simulink model "BMS"  (R2024b)
settings: Solver=ode23tb  StartTime=0.0  StopTime=1  RelTol=1e-3  EnableMultiTasking=on
PreLoadFcn:
  | % Data of Solar Panel
  | %5000[W]/130[W]
  | % Total power generated by solar panel reaches 5[KW].
  | % each solar panel generates power 130[kW].
  | V = [0    40 80 120 160 180 200 217 240 260 280];
  | I = 5000/130*[0.68 0.675 0.67 0.665 0.660 0.655 0.640 0.6 0.48 0.28 0];
  | 
  | %subplot(211);plot(V,I);xlabel('Voltage[V]');ylabel('Current[a]')
  | %subplot(212);plot(V.*I);title('Power[W]')
  | 
  | % Sample Time[s]
  | Ts =5e-6;
  | 
  | 
  | %MPPT + PV Control
  | % PI control pamameter of Voltage control(Outer loop)
  | Kp_V = 50e-3;
  | Ki_V = 10;
  | 
  | % PI Control pamameter of Current control(Inner loop)
  | Kp_I = 25e-3;
  | Ki_I = 10;
  | 
  | % Utility Interconnection Control
  | % PI Control pamameter of Voltage control(Outer loop)
  | Kp_V2 = 0.01;
  | Ki_V2 = 25;
  | 
  | % PI control pamameter of Current control(Inner loop)
  | Kp_I2 = 0.01;
  | Ki_I2 = 25;
  | 
  | 
  | % Difference of voltege using in MPPT
  | dV = 0.5;
  | 
  | % Battery Control
  | % PI Control pamameter of Voltage control(Outer loop)
  | Kp_VB = 0.4;
  | Ki_VB = 2;
  | 
  | % PI control pamameter of Current control(Inner loop)
  | Kp_IB = 0.1;
  | Ki_IB = 0.5;
undefined symbols (not defined in the file): Acid, Ion, Lead, Lithium, sigbuilder_block
libraries: spsBreakerLib x120, spsBatteryLib x111, spsSeriesRLCBranchLib x59, spsVoltageMeasurementLib x17, spsIdealSwitchLib x15, spsMosfetLib x11, slpidlib x9, spsCurrentMeasurementLib x7, spsPWMGeneratorDCDCLib x7, spsDiodeLib x6, spsPWMGenerator2LevelLib x5, spspowerguiLib x3
(part 5 of 6)

== matlab function BMS/Subsystem18/Swapping battery controller/MATLAB Function7 ==
  settings: updateMethod=DISCRETE
  data: SOC input; LoadOn output; ChargingOn output
function [LoadOn, ChargingOn] = chargeDischargeNode(SOC)
    % This function determines the charging and discharging states
    % based on the state of charge (SOC) of the battery.
    % Inputs:
    %   SOC - Current state of charge (0 to 100)
    % Outputs:
    %   LoadOn - Indicator if the load is on (1) or off (0)
    %   ChargingOn - Indicator if charging is active (1) or not (0)

    % Initialize persistent variables to retain state across function calls
    persistent LoadOnPersistent;
    persistent ChargingOnPersistent;

    if isempty(LoadOnPersistent)  % Initialize on first call
        LoadOnPersistent = 1;     % Load is initially on
        ChargingOnPersistent = 0;  % Charging is initially off
    end

    % Logic for charging and discharging based on SOC levels
    if SOC > 80
        LoadOnPersistent = 1;      % Turn load on if SOC is above 80%
        ChargingOnPersistent = 0;   % Turn charging off
    elseif SOC < 40
        LoadOnPersistent = 0;      % Turn load off if SOC is below 40%
        ChargingOnPersistent = 1;   % Start charging
    end

    % Assign output values from persistent variables
    LoadOn = LoadOnPersistent;
    ChargingOn = ChargingOnPersistent;
end

== matlab function BMS/Subsystem18/Swapping battery controller/MATLAB Function8 ==
  settings: updateMethod=DISCRETE
  data: SOC input; LoadOn output; ChargingOn output
function [LoadOn, ChargingOn] = chargeDischargeNode(SOC)
    % This function determines the charging and discharging states
    % based on the state of charge (SOC) of the battery.
    % Inputs:
    %   SOC - Current state of charge (0 to 100)
    % Outputs:
    %   LoadOn - Indicator if the load is on (1) or off (0)
    %   ChargingOn - Indicator if charging is active (1) or not (0)

    % Initialize persistent variables to retain state across function calls
    persistent LoadOnPersistent;
    persistent ChargingOnPersistent;

    if isempty(LoadOnPersistent)  % Initialize on first call
        LoadOnPersistent = 1;     % Load is initially on
        ChargingOnPersistent = 0;  % Charging is initially off
    end

    % Logic for charging and discharging based on SOC levels
    if SOC > 80
        LoadOnPersistent = 1;      % Turn load on if SOC is above 80%
        ChargingOnPersistent = 0;   % Turn charging off
    elseif SOC < 40
        LoadOnPersistent = 0;      % Turn load off if SOC is below 40%
        ChargingOnPersistent = 1;   % Start charging
    end

    % Assign output values from persistent variables
    LoadOn = LoadOnPersistent;
    ChargingOn = ChargingOnPersistent;
end

== matlab function BMS/Subsystem18/Swapping battery controller/MATLAB Function9 ==
  settings: updateMethod=DISCRETE
  data: SOC input; LoadOn output; ChargingOn output
function [LoadOn, ChargingOn] = chargeDischargeNode(SOC)
    % This function determines the charging and discharging states
    % based on the state of charge (SOC) of the battery.
    % Inputs:
    %   SOC - Current state of charge (0 to 100)
    % Outputs:
    %   LoadOn - Indicator if the load is on (1) or off (0)
    %   ChargingOn - Indicator if charging is active (1) or not (0)

    % Initialize persistent variables to retain state across function calls
    persistent LoadOnPersistent;
    persistent ChargingOnPersistent;

    if isempty(LoadOnPersistent)  % Initialize on first call
        LoadOnPersistent = 1;     % Load is initially on
        ChargingOnPersistent = 0;  % Charging is initially off
    end

    % Logic for charging and discharging based on SOC levels
    if SOC > 80
        LoadOnPersistent = 1;      % Turn load on if SOC is above 80%
        ChargingOnPersistent = 0;   % Turn charging off
    elseif SOC < 40
        LoadOnPersistent = 0;      % Turn load off if SOC is below 40%
        ChargingOnPersistent = 1;   % Start charging
    end

    % Assign output values from persistent variables
    LoadOn = LoadOnPersistent;
    ChargingOn = ChargingOnPersistent;
end

== matlab function BMS/Subsystem18/Swapping battery controller/MATLAB Function10 ==
  settings: updateMethod=DISCRETE
  data: SOC input; LoadOn output; ChargingOn output
function [LoadOn, ChargingOn] = chargeDischargeNode(SOC)
    % This function determines the charging and discharging states
    % based on the state of charge (SOC) of the battery.
    % Inputs:
    %   SOC - Current state of charge (0 to 100)
    % Outputs:
    %   LoadOn - Indicator if the load is on (1) or off (0)
    %   ChargingOn - Indicator if charging is active (1) or not (0)

    % Initialize persistent variables to retain state across function calls
    persistent LoadOnPersistent;
    persistent ChargingOnPersistent;

    if isempty(LoadOnPersistent)  % Initialize on first call
        LoadOnPersistent = 1;     % Load is initially on
        ChargingOnPersistent = 0;  % Charging is initially off
    end

    % Logic for charging and discharging based on SOC levels
    if SOC > 80
        LoadOnPersistent = 1;      % Turn load on if SOC is above 80%
        ChargingOnPersistent = 0;   % Turn charging off
    elseif SOC < 40
        LoadOnPersistent = 0;      % Turn load off if SOC is below 40%
        ChargingOnPersistent = 1;   % Start charging
    end

    % Assign output values from persistent variables
    LoadOn = LoadOnPersistent;
    ChargingOn = ChargingOnPersistent;
end

== matlab function BMS/Subsystem18/Swapping battery controller/MATLAB Function11 ==
  settings: updateMethod=DISCRETE
  data: SOC input; LoadOn output; ChargingOn output
function [LoadOn, ChargingOn] = chargeDischargeNode(SOC)
    % This function determines the charging and discharging states
    % based on the state of charge (SOC) of the battery.
    % Inputs:
    %   SOC - Current state of charge (0 to 100)
    % Outputs:
    %   LoadOn - Indicator if the load is on (1) or off (0)
    %   ChargingOn - Indicator if charging is active (1) or not (0)

    % Initialize persistent variables to retain state across function calls
    persistent LoadOnPersistent;
    persistent ChargingOnPersistent;

    if isempty(LoadOnPersistent)  % Initialize on first call
        LoadOnPersistent = 1;     % Load is initially on
        ChargingOnPersistent = 0;  % Charging is initially off
    end

    % Logic for charging and discharging based on SOC levels
    if SOC > 80
        LoadOnPersistent = 1;      % Turn load on if SOC is above 80%
        ChargingOnPersistent = 0;   % Turn charging off
    elseif SOC < 40
        LoadOnPersistent = 0;      % Turn load off if SOC is below 40%
        ChargingOnPersistent = 1;   % Start charging
    end

    % Assign output values from persistent variables
    LoadOn = LoadOnPersistent;
    ChargingOn = ChargingOnPersistent;
end

== matlab function BMS/Subsystem18/Swapping battery controller/MATLAB Function12 ==
  settings: updateMethod=DISCRETE
  data: SOC input; LoadOn output; ChargingOn output
function [LoadOn, ChargingOn] = chargeDischargeNode(SOC)
    % This function determines the charging and discharging states
    % based on the state of charge (SOC) of the battery.
    % Inputs:
    %   SOC - Current state of charge (0 to 100)
    % Outputs:
    %   LoadOn - Indicator if the load is on (1) or off (0)
    %   ChargingOn - Indicator if charging is active (1) or not (0)

    % Initialize persistent variables to retain state across function calls
    persistent LoadOnPersistent;
    persistent ChargingOnPersistent;

    if isempty(LoadOnPersistent)  % Initialize on first call
        LoadOnPersistent = 1;     % Load is initially on
        ChargingOnPersistent = 0;  % Charging is initially off
    end

    % Logic for charging and discharging based on SOC levels
    if SOC > 80
        LoadOnPersistent = 1;      % Turn load on if SOC is above 80%
        ChargingOnPersistent = 0;   % Turn charging off
    elseif SOC < 40
        LoadOnPersistent = 0;      % Turn load off if SOC is below 40%
        ChargingOnPersistent = 1;   % Start charging
    end

    % Assign output values from persistent variables
    LoadOn = LoadOnPersistent;
    ChargingOn = ChargingOnPersistent;
end

== matlab function BMS/Subsystem18/Swapping battery controller/MATLAB Function13 ==
  settings: updateMethod=DISCRETE
  data: SOC input; LoadOn output; ChargingOn output
function [LoadOn, ChargingOn] = chargeDischargeNode(SOC)
    % This function determines the charging and discharging states
    % based on the state of charge (SOC) of the battery.
    % Inputs:
    %   SOC - Current state of charge (0 to 100)
    % Outputs:
    %   LoadOn - Indicator if the load is on (1) or off (0)
    %   ChargingOn - Indicator if charging is active (1) or not (0)

    % Initialize persistent variables to retain state across function calls
    persistent LoadOnPersistent;
    persistent ChargingOnPersistent;

    if isempty(LoadOnPersistent)  % Initialize on first call
        LoadOnPersistent = 1;     % Load is initially on
        ChargingOnPersistent = 0;  % Charging is initially off
    end

    % Logic for charging and discharging based on SOC levels
    if SOC > 80
        LoadOnPersistent = 1;      % Turn load on if SOC is above 80%
        ChargingOnPersistent = 0;   % Turn charging off
    elseif SOC < 40
        LoadOnPersistent = 0;      % Turn load off if SOC is below 40%
        ChargingOnPersistent = 1;   % Start charging
    end

    % Assign output values from persistent variables
    LoadOn = LoadOnPersistent;
    ChargingOn = ChargingOnPersistent;
end

== matlab function BMS/Subsystem18/Swapping battery controller/MATLAB Function14 ==
  settings: updateMethod=DISCRETE
  data: SOC input; LoadOn output; ChargingOn output
function [LoadOn, ChargingOn] = chargeDischargeNode(SOC)
    % This function determines the charging and discharging states
    % based on the state of charge (SOC) of the battery.
    % Inputs:
    %   SOC - Current state of charge (0 to 100)
    % Outputs:
    %   LoadOn - Indicator if the load is on (1) or off (0)
    %   ChargingOn - Indicator if charging is active (1) or not (0)

    % Initialize persistent variables to retain state across function calls
    persistent LoadOnPersistent;
    persistent ChargingOnPersistent;

    if isempty(LoadOnPersistent)  % Initialize on first call
        LoadOnPersistent = 1;     % Load is initially on
        ChargingOnPersistent = 0;  % Charging is initially off
    end

    % Logic for charging and discharging based on SOC levels
    if SOC > 80
        LoadOnPersistent = 1;      % Turn load on if SOC is above 80%
        ChargingOnPersistent = 0;   % Turn charging off
    elseif SOC < 40
        LoadOnPersistent = 0;      % Turn load off if SOC is below 40%
        ChargingOnPersistent = 1;   % Start charging
    end

    % Assign output values from persistent variables
    LoadOn = LoadOnPersistent;
    ChargingOn = ChargingOnPersistent;
end

== matlab function BMS/Subsystem18/Swapping battery controller/MATLAB Function15 ==
  settings: updateMethod=DISCRETE
  data: SOC input; LoadOn output; ChargingOn output
function [LoadOn, ChargingOn] = chargeDischargeNode(SOC)
    % This function determines the charging and discharging states
    % based on the state of charge (SOC) of the battery.
    % Inputs:
    %   SOC - Current state of charge (0 to 100)
    % Outputs:
    %   LoadOn - Indicator if the load is on (1) or off (0)
    %   ChargingOn - Indicator if charging is active (1) or not (0)

    % Initialize persistent variables to retain state across function calls
    persistent LoadOnPersistent;
    persistent ChargingOnPersistent;

    if isempty(LoadOnPersistent)  % Initialize on first call
        LoadOnPersistent = 1;     % Load is initially on
        ChargingOnPersistent = 0;  % Charging is initially off
    end

    % Logic for charging and discharging based on SOC levels
    if SOC > 80
        LoadOnPersistent = 1;      % Turn load on if SOC is above 80%
        ChargingOnPersistent = 0;   % Turn charging off
    elseif SOC < 40
        LoadOnPersistent = 0;      % Turn load off if SOC is below 40%
        ChargingOnPersistent = 1;   % Start charging
    end

    % Assign output values from persistent variables
    LoadOn = LoadOnPersistent;
    ChargingOn = ChargingOnPersistent;
end

== matlab function BMS/Subsystem18/Swapping battery controller/MATLAB Function16 ==
  settings: updateMethod=DISCRETE
  data: SOC input; LoadOn output; ChargingOn output
function [LoadOn, ChargingOn] = chargeDischargeNode(SOC)
    % This function determines the charging and discharging states
    % based on the state of charge (SOC) of the battery.
    % Inputs:
    %   SOC - Current state of charge (0 to 100)
    % Outputs:
    %   LoadOn - Indicator if the load is on (1) or off (0)
    %   ChargingOn - Indicator if charging is active (1) or not (0)

    % Initialize persistent variables to retain state across function calls
    persistent LoadOnPersistent;
    persistent ChargingOnPersistent;

    if isempty(LoadOnPersistent)  % Initialize on first call
        LoadOnPersistent = 1;     % Load is initially on
        ChargingOnPersistent = 0;  % Charging is initially off
    end

    % Logic for charging and discharging based on SOC levels
    if SOC > 80
        LoadOnPersistent = 1;      % Turn load on if SOC is above 80%
        ChargingOnPersistent = 0;   % Turn charging off
    elseif SOC < 40
        LoadOnPersistent = 0;      % Turn load off if SOC is below 40%
        ChargingOnPersistent = 1;   % Start charging
    end

    % Assign output values from persistent variables
    LoadOn = LoadOnPersistent;
    ChargingOn = ChargingOnPersistent;
end

== matlab function BMS/Subsystem18/Swapping battery controller/MATLAB Function17 ==
  settings: updateMethod=DISCRETE
  data: SOC input; LoadOn output; ChargingOn output
function [LoadOn, ChargingOn] = chargeDischargeNode(SOC)
    % This function determines the charging and discharging states
    % based on the state of charge (SOC) of the battery.
    % Inputs:
    %   SOC - Current state of charge (0 to 100)
    % Outputs:
    %   LoadOn - Indicator if the load is on (1) or off (0)
    %   ChargingOn - Indicator if charging is active (1) or not (0)

    % Initialize persistent variables to retain state across function calls
    persistent LoadOnPersistent;
    persistent ChargingOnPersistent;

    if isempty(LoadOnPersistent)  % Initialize on first call
        LoadOnPersistent = 1;     % Load is initially on
        ChargingOnPersistent = 0;  % Charging is initially off
    end

    % Logic for charging and discharging based on SOC levels
    if SOC > 80
        LoadOnPersistent = 1;      % Turn load on if SOC is above 80%
        ChargingOnPersistent = 0;   % Turn charging off
    elseif SOC < 40
        LoadOnPersistent = 0;      % Turn load off if SOC is below 40%
        ChargingOnPersistent = 1;   % Start charging
    end

    % Assign output values from persistent variables
    LoadOn = LoadOnPersistent;
    ChargingOn = ChargingOnPersistent;
end

== matlab function BMS/Subsystem18/Swapping battery controller/MATLAB Function18 ==
  settings: updateMethod=DISCRETE
  data: SOC input; LoadOn output; ChargingOn output
function [LoadOn, ChargingOn] = chargeDischargeNode(SOC)
    % This function determines the charging and discharging states
    % based on the state of charge (SOC) of the battery.
    % Inputs:
    %   SOC - Current state of charge (0 to 100)
    % Outputs:
    %   LoadOn - Indicator if the load is on (1) or off (0)
    %   ChargingOn - Indicator if charging is active (1) or not (0)

    % Initialize persistent variables to retain state across function calls
    persistent LoadOnPersistent;
    persistent ChargingOnPersistent;

    if isempty(LoadOnPersistent)  % Initialize on first call
        LoadOnPersistent = 1;     % Load is initially on
        ChargingOnPersistent = 0;  % Charging is initially off
    end

    % Logic for charging and discharging based on SOC levels
    if SOC > 80
        LoadOnPersistent = 1;      % Turn load on if SOC is above 80%
        ChargingOnPersistent = 0;   % Turn charging off
    elseif SOC < 40
        LoadOnPersistent = 0;      % Turn load off if SOC is below 40%
        ChargingOnPersistent = 1;   % Start charging
    end

    % Assign output values from persistent variables
    LoadOn = LoadOnPersistent;
    ChargingOn = ChargingOnPersistent;
end

== matlab function BMS/Subsystem18/Swapping battery controller/MATLAB Function19 ==
  settings: updateMethod=DISCRETE
  data: SOC input; LoadOn output; ChargingOn output
function [LoadOn, ChargingOn] = chargeDischargeNode(SOC)
    % This function determines the charging and discharging states
    % based on the state of charge (SOC) of the battery.
    % Inputs:
    %   SOC - Current state of charge (0 to 100)
    % Outputs:
    %   LoadOn - Indicator if the load is on (1) or off (0)
    %   ChargingOn - Indicator if charging is active (1) or not (0)

    % Initialize persistent variables to retain state across function calls
    persistent LoadOnPersistent;
    persistent ChargingOnPersistent;

    if isempty(LoadOnPersistent)  % Initialize on first call
        LoadOnPersistent = 1;     % Load is initially on
        ChargingOnPersistent = 0;  % Charging is initially off
    end

    % Logic for charging and discharging based on SOC levels
    if SOC > 80
        LoadOnPersistent = 1;      % Turn load on if SOC is above 80%
        ChargingOnPersistent = 0;   % Turn charging off
    elseif SOC < 40
        LoadOnPersistent = 0;      % Turn load off if SOC is below 40%
        ChargingOnPersistent = 1;   % Start charging
    end

    % Assign output values from persistent variables
    LoadOn = LoadOnPersistent;
    ChargingOn = ChargingOnPersistent;
end

== matlab function BMS/Subsystem18/Swapping battery controller/MATLAB Function20 ==
  settings: updateMethod=DISCRETE
  data: SOC input; LoadOn output; ChargingOn output
function [LoadOn, ChargingOn] = chargeDischargeNode(SOC)
    % This function determines the charging and discharging states
    % based on the state of charge (SOC) of the battery.
    % Inputs:
    %   SOC - Current state of charge (0 to 100)
    % Outputs:
    %   LoadOn - Indicator if the load is on (1) or off (0)
    %   ChargingOn - Indicator if charging is active (1) or not (0)

    % Initialize persistent variables to retain state across function calls
    persistent LoadOnPersistent;
    persistent ChargingOnPersistent;

    if isempty(LoadOnPersistent)  % Initialize on first call
        LoadOnPersistent = 1;     % Load is initially on
        ChargingOnPersistent = 0;  % Charging is initially off
    end

    % Logic for charging and discharging based on SOC levels
    if SOC > 80
        LoadOnPersistent = 1;      % Turn load on if SOC is above 80%
        ChargingOnPersistent = 0;   % Turn charging off
    elseif SOC < 40
        LoadOnPersistent = 0;      % Turn load off if SOC is below 40%
        ChargingOnPersistent = 1;   % Start charging
    end

    % Assign output values from persistent variables
    LoadOn = LoadOnPersistent;
    ChargingOn = ChargingOnPersistent;
end

== matlab function BMS/Subsystem18/Swapping battery controller/MATLAB Function21 ==
  settings: updateMethod=DISCRETE
  data: SOC input; LoadOn output; ChargingOn output
function [LoadOn, ChargingOn] = chargeDischargeNode(SOC)
    % This function determines the charging and discharging states
    % based on the state of charge (SOC) of the battery.
    % Inputs:
    %   SOC - Current state of charge (0 to 100)
    % Outputs:
    %   LoadOn - Indicator if the load is on (1) or off (0)
    %   ChargingOn - Indicator if charging is active (1) or not (0)

    % Initialize persistent variables to retain state across function calls
    persistent LoadOnPersistent;
    persistent ChargingOnPersistent;

    if isempty(LoadOnPersistent)  % Initialize on first call
        LoadOnPersistent = 1;     % Load is initially on
        ChargingOnPersistent = 0;  % Charging is initially off
    end

    % Logic for charging and discharging based on SOC levels
    if SOC > 80
        LoadOnPersistent = 1;      % Turn load on if SOC is above 80%
        ChargingOnPersistent = 0;   % Turn charging off
    elseif SOC < 40
        LoadOnPersistent = 0;      % Turn load off if SOC is below 40%
        ChargingOnPersistent = 1;   % Start charging
    end

    % Assign output values from persistent variables
    LoadOn = LoadOnPersistent;
    ChargingOn = ChargingOnPersistent;
end

== matlab function BMS/Subsystem18/Swapping battery controller/MATLAB Function22 ==
  settings: updateMethod=DISCRETE
  data: SOC input; LoadOn output; ChargingOn output
function [LoadOn, ChargingOn] = chargeDischargeNode(SOC)
    % This function determines the charging and discharging states
    % based on the state of charge (SOC) of the battery.
    % Inputs:
    %   SOC - Current state of charge (0 to 100)
    % Outputs:
    %   LoadOn - Indicator if the load is on (1) or off (0)
    %   ChargingOn - Indicator if charging is active (1) or not (0)

    % Initialize persistent variables to retain state across function calls
    persistent LoadOnPersistent;
    persistent ChargingOnPersistent;

    if isempty(LoadOnPersistent)  % Initialize on first call
        LoadOnPersistent = 1;     % Load is initially on
        ChargingOnPersistent = 0;  % Charging is initially off
    end

    % Logic for charging and discharging based on SOC levels
    if SOC > 80
        LoadOnPersistent = 1;      % Turn load on if SOC is above 80%
        ChargingOnPersistent = 0;   % Turn charging off
    elseif SOC < 40
        LoadOnPersistent = 0;      % Turn load off if SOC is below 40%
        ChargingOnPersistent = 1;   % Start charging
    end

    % Assign output values from persistent variables
    LoadOn = LoadOnPersistent;
    ChargingOn = ChargingOnPersistent;
end

== matlab function BMS/Subsystem18/Swapping battery controller/MATLAB Function23 ==
  settings: updateMethod=DISCRETE
  data: SOC input; LoadOn output; ChargingOn output
function [LoadOn, ChargingOn] = chargeDischargeNode(SOC)
    % This function determines the charging and discharging states
    % based on the state of charge (SOC) of the battery.
    % Inputs:
    %   SOC - Current state of charge (0 to 100)
    % Outputs:
    %   LoadOn - Indicator if the load is on (1) or off (0)
    %   ChargingOn - Indicator if charging is active (1) or not (0)

    % Initialize persistent variables to retain state across function calls
    persistent LoadOnPersistent;
    persistent ChargingOnPersistent;

    if isempty(LoadOnPersistent)  % Initialize on first call
        LoadOnPersistent = 1;     % Load is initially on
        ChargingOnPersistent = 0;  % Charging is initially off
    end

    % Logic for charging and discharging based on SOC levels
    if SOC > 80
        LoadOnPersistent = 1;      % Turn load on if SOC is above 80%
        ChargingOnPersistent = 0;   % Turn charging off
    elseif SOC < 40
        LoadOnPersistent = 0;      % Turn load off if SOC is below 40%
        ChargingOnPersistent = 1;   % Start charging
    end

    % Assign output values from persistent variables
    LoadOn = LoadOnPersistent;
    ChargingOn = ChargingOnPersistent;
end

== matlab function BMS/Subsystem18/Swapping battery controller/MATLAB Function24 ==
  settings: updateMethod=DISCRETE
  data: SOC input; LoadOn output; ChargingOn output
function [LoadOn, ChargingOn] = chargeDischargeNode(SOC)
    % This function determines the charging and discharging states
    % based on the state of charge (SOC) of the battery.
    % Inputs:
    %   SOC - Current state of charge (0 to 100)
    % Outputs:
    %   LoadOn - Indicator if the load is on (1) or off (0)
    %   ChargingOn - Indicator if charging is active (1) or not (0)

    % Initialize persistent variables to retain state across function calls
    persistent LoadOnPersistent;
    persistent ChargingOnPersistent;

    if isempty(LoadOnPersistent)  % Initialize on first call
        LoadOnPersistent = 1;     % Load is initially on
        ChargingOnPersistent = 0;  % Charging is initially off
    end

    % Logic for charging and discharging based on SOC levels
    if SOC > 80
        LoadOnPersistent = 1;      % Turn load on if SOC is above 80%
        ChargingOnPersistent = 0;   % Turn charging off
    elseif SOC < 40
        LoadOnPersistent = 0;      % Turn load off if SOC is below 40%
        ChargingOnPersistent = 1;   % Start charging
    end

    % Assign output values from persistent variables
    LoadOn = LoadOnPersistent;
    ChargingOn = ChargingOnPersistent;
end

== matlab function BMS/Subsystem18/Swapping battery controller/MATLAB Function25 ==
  settings: updateMethod=DISCRETE
  data: SOC input; LoadOn output; ChargingOn output
function [LoadOn, ChargingOn] = chargeDischargeNode(SOC)
    % This function determines the charging and discharging states
    % based on the state of charge (SOC) of the battery.
    % Inputs:
    %   SOC - Current state of charge (0 to 100)
    % Outputs:
    %   LoadOn - Indicator if the load is on (1) or off (0)
    %   ChargingOn - Indicator if charging is active (1) or not (0)

    % Initialize persistent variables to retain state across function calls
    persistent LoadOnPersistent;
    persistent ChargingOnPersistent;

    if isempty(LoadOnPersistent)  % Initialize on first call
        LoadOnPersistent = 1;     % Load is initially on
        ChargingOnPersistent = 0;  % Charging is initially off
    end

    % Logic for charging and discharging based on SOC levels
    if SOC > 80
        LoadOnPersistent = 1;      % Turn load on if SOC is above 80%
        ChargingOnPersistent = 0;   % Turn charging off
    elseif SOC < 40
        LoadOnPersistent = 0;      % Turn load off if SOC is below 40%
        ChargingOnPersistent = 1;   % Start charging
    end

    % Assign output values from persistent variables
    LoadOn = LoadOnPersistent;
    ChargingOn = ChargingOnPersistent;
end

== matlab function BMS/Subsystem18/Swapping battery controller/MATLAB Function26 ==
  settings: updateMethod=DISCRETE
  data: SOC input; LoadOn output; ChargingOn output
function [LoadOn, ChargingOn] = chargeDischargeNode(SOC)
    % This function determines the charging and discharging states
    % based on the state of charge (SOC) of the battery.
    % Inputs:
    %   SOC - Current state of charge (0 to 100)
    % Outputs:
    %   LoadOn - Indicator if the load is on (1) or off (0)
    %   ChargingOn - Indicator if charging is active (1) or not (0)

    % Initialize persistent variables to retain state across function calls
    persistent LoadOnPersistent;
    persistent ChargingOnPersistent;

    if isempty(LoadOnPersistent)  % Initialize on first call
        LoadOnPersistent = 1;     % Load is initially on
        ChargingOnPersistent = 0;  % Charging is initially off
    end

    % Logic for charging and discharging based on SOC levels
    if SOC > 80
        LoadOnPersistent = 1;      % Turn load on if SOC is above 80%
        ChargingOnPersistent = 0;   % Turn charging off
    elseif SOC < 40
        LoadOnPersistent = 0;      % Turn load off if SOC is below 40%
        ChargingOnPersistent = 1;   % Start charging
    end

    % Assign output values from persistent variables
    LoadOn = LoadOnPersistent;
    ChargingOn = ChargingOnPersistent;
end

== matlab function BMS/Subsystem18/Swapping battery controller/MATLAB Function27 ==
  settings: updateMethod=DISCRETE
  data: SOC input; LoadOn output; ChargingOn output
function [LoadOn, ChargingOn] = chargeDischargeNode(SOC)
    % This function determines the charging and discharging states
    % based on the state of charge (SOC) of the battery.
    % Inputs:
    %   SOC - Current state of charge (0 to 100)
    % Outputs:
    %   LoadOn - Indicator if the load is on (1) or off (0)
    %   ChargingOn - Indicator if charging is active (1) or not (0)

    % Initialize persistent variables to retain state across function calls
    persistent LoadOnPersistent;
    persistent ChargingOnPersistent;

    if isempty(LoadOnPersistent)  % Initialize on first call
        LoadOnPersistent = 1;     % Load is initially on
        ChargingOnPersistent = 0;  % Charging is initially off
    end

    % Logic for charging and discharging based on SOC levels
    if SOC > 80
        LoadOnPersistent = 1;      % Turn load on if SOC is above 80%
        ChargingOnPersistent = 0;   % Turn charging off
    elseif SOC < 40
        LoadOnPersistent = 0;      % Turn load off if SOC is below 40%
        ChargingOnPersistent = 1;   % Start charging
    end

    % Assign output values from persistent variables
    LoadOn = LoadOnPersistent;
    ChargingOn = ChargingOnPersistent;
end

== matlab function BMS/Subsystem18/Swapping battery controller/MATLAB Function28 ==
  settings: updateMethod=DISCRETE
  data: SOC input; LoadOn output; ChargingOn output
function [LoadOn, ChargingOn] = chargeDischargeNode(SOC)
    % This function determines the charging and discharging states
    % based on the state of charge (SOC) of the battery.
    % Inputs:
    %   SOC - Current state of charge (0 to 100)
    % Outputs:
    %   LoadOn - Indicator if the load is on (1) or off (0)
    %   ChargingOn - Indicator if charging is active (1) or not (0)

    % Initialize persistent variables to retain state across function calls
    persistent LoadOnPersistent;
    persistent ChargingOnPersistent;

    if isempty(LoadOnPersistent)  % Initialize on first call
        LoadOnPersistent = 1;     % Load is initially on
        ChargingOnPersistent = 0;  % Charging is initially off
    end

    % Logic for charging and discharging based on SOC levels
    if SOC > 80
        LoadOnPersistent = 1;      % Turn load on if SOC is above 80%
        ChargingOnPersistent = 0;   % Turn charging off
    elseif SOC < 40
        LoadOnPersistent = 0;      % Turn load off if SOC is below 40%
        ChargingOnPersistent = 1;   % Start charging
    end

    % Assign output values from persistent variables
    LoadOn = LoadOnPersistent;
    ChargingOn = ChargingOnPersistent;
end

== matlab function BMS/Subsystem18/Swapping battery controller/MATLAB Function29 ==
  settings: updateMethod=DISCRETE
  data: SOC input; LoadOn output; ChargingOn output
function [LoadOn, ChargingOn] = chargeDischargeNode(SOC)
    % This function determines the charging and discharging states
    % based on the state of charge (SOC) of the battery.
    % Inputs:
    %   SOC - Current state of charge (0 to 100)
    % Outputs:
    %   LoadOn - Indicator if the load is on (1) or off (0)
    %   ChargingOn - Indicator if charging is active (1) or not (0)

    % Initialize persistent variables to retain state across function calls
    persistent LoadOnPersistent;
    persistent ChargingOnPersistent;

    if isempty(LoadOnPersistent)  % Initialize on first call
        LoadOnPersistent = 1;     % Load is initially on
        ChargingOnPersistent = 0;  % Charging is initially off
    end

    % Logic for charging and discharging based on SOC levels
    if SOC > 80
        LoadOnPersistent = 1;      % Turn load on if SOC is above 80%
        ChargingOnPersistent = 0;   % Turn charging off
    elseif SOC < 40
        LoadOnPersistent = 0;      % Turn load off if SOC is below 40%
        ChargingOnPersistent = 1;   % Start charging
    end

    % Assign output values from persistent variables
    LoadOn = LoadOnPersistent;
    ChargingOn = ChargingOnPersistent;
end

== matlab function BMS/MPPT and PV Controller/Swapping battery controller/MATLAB Function ==
  settings: updateMethod=DISCRETE
  data: SOC input; LoadOn output; ChargingOn output
function [LoadOn, ChargingOn] = chargeDischargeNode(SOC)
    % This function determines the charging and discharging states
    % based on the state of charge (SOC) of the battery.
    % Inputs:
    %   SOC - Current state of charge (0 to 100)
    % Outputs:
    %   LoadOn - Indicator if the load is on (1) or off (0)
    %   ChargingOn - Indicator if charging is active (1) or not (0)

    % Initialize persistent variables to retain state across function calls
    persistent LoadOnPersistent;
    persistent ChargingOnPersistent;

    if isempty(LoadOnPersistent)  % Initialize on first call
        LoadOnPersistent = 1;     % Load is initially on
        ChargingOnPersistent = 0;  % Charging is initially off
    end

    % Logic for charging and discharging based on SOC levels
    if SOC > 80
        LoadOnPersistent = 1;      % Turn load on if SOC is above 80%
        ChargingOnPersistent = 0;   % Turn charging off
    elseif SOC < 40
        LoadOnPersistent = 0;      % Turn load off if SOC is below 40%
        ChargingOnPersistent = 1;   % Start charging
    end

    % Assign output values from persistent variables
    LoadOn = LoadOnPersistent;
    ChargingOn = ChargingOnPersistent;
end

== matlab function BMS/MPPT and PV Controller/Swapping battery controller/MATLAB Function1 ==
  settings: updateMethod=DISCRETE
  data: SOC input; LoadOn output; ChargingOn output
function [LoadOn, ChargingOn] = chargeDischargeNode(SOC)
    % This function determines the charging and discharging states
    % based on the state of charge (SOC) of the battery.
    % Inputs:
    %   SOC - Current state of charge (0 to 100)
    % Outputs:
    %   LoadOn - Indicator if the load is on (1) or off (0)
    %   ChargingOn - Indicator if charging is active (1) or not (0)

    % Initialize persistent variables to retain state across function calls
    persistent LoadOnPersistent;
    persistent ChargingOnPersistent;

    if isempty(LoadOnPersistent)  % Initialize on first call
        LoadOnPersistent = 1;     % Load is initially on
        ChargingOnPersistent = 0;  % Charging is initially off
    end

    % Logic for charging and discharging based on SOC levels
    if SOC > 80
        LoadOnPersistent = 1;      % Turn load on if SOC is above 80%
        ChargingOnPersistent = 0;   % Turn charging off
    elseif SOC < 40
        LoadOnPersistent = 0;      % Turn load off if SOC is below 40%
        ChargingOnPersistent = 1;   % Start charging
    end

    % Assign output values from persistent variables
    LoadOn = LoadOnPersistent;
    ChargingOn = ChargingOnPersistent;
end

== matlab function BMS/MPPT and PV Controller/Swapping battery controller/MATLAB Function10 ==
  settings: updateMethod=DISCRETE
  data: SOC input; LoadOn output; ChargingOn output
function [LoadOn, ChargingOn] = chargeDischargeNode(SOC)
    % This function determines the charging and discharging states
    % based on the state of charge (SOC) of the battery.
    % Inputs:
    %   SOC - Current state of charge (0 to 100)
    % Outputs:
    %   LoadOn - Indicator if the load is on (1) or off (0)
    %   ChargingOn - Indicator if charging is active (1) or not (0)

    % Initialize persistent variables to retain state across function calls
    persistent LoadOnPersistent;
    persistent ChargingOnPersistent;

    if isempty(LoadOnPersistent)  % Initialize on first call
        LoadOnPersistent = 1;     % Load is initially on
        ChargingOnPersistent = 0;  % Charging is initially off
    end

    % Logic for charging and discharging based on SOC levels
    if SOC > 80
        LoadOnPersistent = 1;      % Turn load on if SOC is above 80%
        ChargingOnPersistent = 0;   % Turn charging off
    elseif SOC < 40
        LoadOnPersistent = 0;      % Turn load off if SOC is below 40%
        ChargingOnPersistent = 1;   % Start charging
    end

    % Assign output values from persistent variables
    LoadOn = LoadOnPersistent;
    ChargingOn = ChargingOnPersistent;
end

== matlab function BMS/MPPT and PV Controller/Swapping battery controller/MATLAB Function11 ==
  settings: updateMethod=DISCRETE
  data: SOC input; LoadOn output; ChargingOn output
function [LoadOn, ChargingOn] = chargeDischargeNode(SOC)
    % This function determines the charging and discharging states
    % based on the state of charge (SOC) of the battery.
    % Inputs:
    %   SOC - Current state of charge (0 to 100)
    % Outputs:
    %   LoadOn - Indicator if the load is on (1) or off (0)
    %   ChargingOn - Indicator if charging is active (1) or not (0)

    % Initialize persistent variables to retain state across function calls
    persistent LoadOnPersistent;
    persistent ChargingOnPersistent;

    if isempty(LoadOnPersistent)  % Initialize on first call
        LoadOnPersistent = 1;     % Load is initially on
        ChargingOnPersistent = 0;  % Charging is initially off
    end

    % Logic for charging and discharging based on SOC levels
    if SOC > 80
        LoadOnPersistent = 1;      % Turn load on if SOC is above 80%
        ChargingOnPersistent = 0;   % Turn charging off
    elseif SOC < 40
        LoadOnPersistent = 0;      % Turn load off if SOC is below 40%
        ChargingOnPersistent = 1;   % Start charging
    end

    % Assign output values from persistent variables
    LoadOn = LoadOnPersistent;
    ChargingOn = ChargingOnPersistent;
end

== matlab function BMS/MPPT and PV Controller/Swapping battery controller/MATLAB Function12 ==
  settings: updateMethod=DISCRETE
  data: SOC input; LoadOn output; ChargingOn output
function [LoadOn, ChargingOn] = chargeDischargeNode(SOC)
    % This function determines the charging and discharging states
    % based on the state of charge (SOC) of the battery.
    % Inputs:
    %   SOC - Current state of charge (0 to 100)
    % Outputs:
    %   LoadOn - Indicator if the load is on (1) or off (0)
    %   ChargingOn - Indicator if charging is active (1) or not (0)

    % Initialize persistent variables to retain state across function calls
    persistent LoadOnPersistent;
    persistent ChargingOnPersistent;

    if isempty(LoadOnPersistent)  % Initialize on first call
        LoadOnPersistent = 1;     % Load is initially on
        ChargingOnPersistent = 0;  % Charging is initially off
    end

    % Logic for charging and discharging based on SOC levels
    if SOC > 80
        LoadOnPersistent = 1;      % Turn load on if SOC is above 80%
        ChargingOnPersistent = 0;   % Turn charging off
    elseif SOC < 40
        LoadOnPersistent = 0;      % Turn load off if SOC is below 40%
        ChargingOnPersistent = 1;   % Start charging
    end

    % Assign output values from persistent variables
    LoadOn = LoadOnPersistent;
    ChargingOn = ChargingOnPersistent;
end

== matlab function BMS/MPPT and PV Controller/Swapping battery controller/MATLAB Function13 ==
  settings: updateMethod=DISCRETE
  data: SOC input; LoadOn output; ChargingOn output
function [LoadOn, ChargingOn] = chargeDischargeNode(SOC)
    % This function determines the charging and discharging states
    % based on the state of charge (SOC) of the battery.
    % Inputs:
    %   SOC - Current state of charge (0 to 100)
    % Outputs:
    %   LoadOn - Indicator if the load is on (1) or off (0)
    %   ChargingOn - Indicator if charging is active (1) or not (0)

    % Initialize persistent variables to retain state across function calls
    persistent LoadOnPersistent;
    persistent ChargingOnPersistent;

    if isempty(LoadOnPersistent)  % Initialize on first call
        LoadOnPersistent = 1;     % Load is initially on
        ChargingOnPersistent = 0;  % Charging is initially off
    end

    % Logic for charging and discharging based on SOC levels
    if SOC > 80
        LoadOnPersistent = 1;      % Turn load on if SOC is above 80%
        ChargingOnPersistent = 0;   % Turn charging off
    elseif SOC < 40
        LoadOnPersistent = 0;      % Turn load off if SOC is below 40%
        ChargingOnPersistent = 1;   % Start charging
    end

    % Assign output values from persistent variables
    LoadOn = LoadOnPersistent;
    ChargingOn = ChargingOnPersistent;
end

== matlab function BMS/MPPT and PV Controller/Swapping battery controller/MATLAB Function14 ==
  settings: updateMethod=DISCRETE
  data: SOC input; LoadOn output; ChargingOn output
function [LoadOn, ChargingOn] = chargeDischargeNode(SOC)
    % This function determines the charging and discharging states
    % based on the state of charge (SOC) of the battery.
    % Inputs:
    %   SOC - Current state of charge (0 to 100)
    % Outputs:
    %   LoadOn - Indicator if the load is on (1) or off (0)
    %   ChargingOn - Indicator if charging is active (1) or not (0)

    % Initialize persistent variables to retain state across function calls
    persistent LoadOnPersistent;
    persistent ChargingOnPersistent;

    if isempty(LoadOnPersistent)  % Initialize on first call
        LoadOnPersistent = 1;     % Load is initially on
        ChargingOnPersistent = 0;  % Charging is initially off
    end

    % Logic for charging and discharging based on SOC levels
    if SOC > 80
        LoadOnPersistent = 1;      % Turn load on if SOC is above 80%
        ChargingOnPersistent = 0;   % Turn charging off
    elseif SOC < 40
        LoadOnPersistent = 0;      % Turn load off if SOC is below 40%
        ChargingOnPersistent = 1;   % Start charging
    end

    % Assign output values from persistent variables
    LoadOn = LoadOnPersistent;
    ChargingOn = ChargingOnPersistent;
end

== matlab function BMS/MPPT and PV Controller/Swapping battery controller/MATLAB Function15 ==
  settings: updateMethod=DISCRETE
  data: SOC input; LoadOn output; ChargingOn output
function [LoadOn, ChargingOn] = chargeDischargeNode(SOC)
    % This function determines the charging and discharging states
    % based on the state of charge (SOC) of the battery.
    % Inputs:
    %   SOC - Current state of charge (0 to 100)
    % Outputs:
    %   LoadOn - Indicator if the load is on (1) or off (0)
    %   ChargingOn - Indicator if charging is active (1) or not (0)

    % Initialize persistent variables to retain state across function calls
    persistent LoadOnPersistent;
    persistent ChargingOnPersistent;

    if isempty(LoadOnPersistent)  % Initialize on first call
        LoadOnPersistent = 1;     % Load is initially on
        ChargingOnPersistent = 0;  % Charging is initially off
    end

    % Logic for charging and discharging based on SOC levels
    if SOC > 80
        LoadOnPersistent = 1;      % Turn load on if SOC is above 80%
        ChargingOnPersistent = 0;   % Turn charging off
    elseif SOC < 40
        LoadOnPersistent = 0;      % Turn load off if SOC is below 40%
        ChargingOnPersistent = 1;   % Start charging
    end

    % Assign output values from persistent variables
    LoadOn = LoadOnPersistent;
    ChargingOn = ChargingOnPersistent;
end

== matlab function BMS/MPPT and PV Controller/Swapping battery controller/MATLAB Function16 ==
  settings: updateMethod=DISCRETE
  data: SOC input; LoadOn output; ChargingOn output
function [LoadOn, ChargingOn] = chargeDischargeNode(SOC)
    % This function determines the charging and discharging states
    % based on the state of charge (SOC) of the battery.
    % Inputs:
    %   SOC - Current state of charge (0 to 100)
    % Outputs:
    %   LoadOn - Indicator if the load is on (1) or off (0)
    %   ChargingOn - Indicator if charging is active (1) or not (0)

    % Initialize persistent variables to retain state across function calls
    persistent LoadOnPersistent;
    persistent ChargingOnPersistent;

    if isempty(LoadOnPersistent)  % Initialize on first call
        LoadOnPersistent = 1;     % Load is initially on
        ChargingOnPersistent = 0;  % Charging is initially off
    end

    % Logic for charging and discharging based on SOC levels
    if SOC > 80
        LoadOnPersistent = 1;      % Turn load on if SOC is above 80%
        ChargingOnPersistent = 0;   % Turn charging off
    elseif SOC < 40
        LoadOnPersistent = 0;      % Turn load off if SOC is below 40%
        ChargingOnPersistent = 1;   % Start charging
    end

    % Assign output values from persistent variables
    LoadOn = LoadOnPersistent;
    ChargingOn = ChargingOnPersistent;
end

== matlab function BMS/MPPT and PV Controller/Swapping battery controller/MATLAB Function17 ==
  settings: updateMethod=DISCRETE
  data: SOC input; LoadOn output; ChargingOn output
function [LoadOn, ChargingOn] = chargeDischargeNode(SOC)
    % This function determines the charging and discharging states
    % based on the state of charge (SOC) of the battery.
    % Inputs:
    %   SOC - Current state of charge (0 to 100)
    % Outputs:
    %   LoadOn - Indicator if the load is on (1) or off (0)
    %   ChargingOn - Indicator if charging is active (1) or not (0)

    % Initialize persistent variables to retain state across function calls
    persistent LoadOnPersistent;
    persistent ChargingOnPersistent;

    if isempty(LoadOnPersistent)  % Initialize on first call
        LoadOnPersistent = 1;     % Load is initially on
        ChargingOnPersistent = 0;  % Charging is initially off
    end

    % Logic for charging and discharging based on SOC levels
    if SOC > 80
        LoadOnPersistent = 1;      % Turn load on if SOC is above 80%
        ChargingOnPersistent = 0;   % Turn charging off
    elseif SOC < 40
        LoadOnPersistent = 0;      % Turn load off if SOC is below 40%
        ChargingOnPersistent = 1;   % Start charging
    end

    % Assign output values from persistent variables
    LoadOn = LoadOnPersistent;
    ChargingOn = ChargingOnPersistent;
end

== matlab function BMS/MPPT and PV Controller/Swapping battery controller/MATLAB Function18 ==
  settings: updateMethod=DISCRETE
  data: SOC input; LoadOn output; ChargingOn output
function [LoadOn, ChargingOn] = chargeDischargeNode(SOC)
    % This function determines the charging and discharging states
    % based on the state of charge (SOC) of the battery.
    % Inputs:
    %   SOC - Current state of charge (0 to 100)
    % Outputs:
    %   LoadOn - Indicator if the load is on (1) or off (0)
    %   ChargingOn - Indicator if charging is active (1) or not (0)

    % Initialize persistent variables to retain state across function calls
    persistent LoadOnPersistent;
    persistent ChargingOnPersistent;

    if isempty(LoadOnPersistent)  % Initialize on first call
        LoadOnPersistent = 1;     % Load is initially on
        ChargingOnPersistent = 0;  % Charging is initially off
    end

    % Logic for charging and discharging based on SOC levels
    if SOC > 80
        LoadOnPersistent = 1;      % Turn load on if SOC is above 80%
        ChargingOnPersistent = 0;   % Turn charging off
    elseif SOC < 40
        LoadOnPersistent = 0;      % Turn load off if SOC is below 40%
        ChargingOnPersistent = 1;   % Start charging
    end

    % Assign output values from persistent variables
    LoadOn = LoadOnPersistent;
    ChargingOn = ChargingOnPersistent;
end

== matlab function BMS/MPPT and PV Controller/Swapping battery controller/MATLAB Function19 ==
  settings: updateMethod=DISCRETE
  data: SOC input; LoadOn output; ChargingOn output
function [LoadOn, ChargingOn] = chargeDischargeNode(SOC)
    % This function determines the charging and discharging states
    % based on the state of charge (SOC) of the battery.
    % Inputs:
    %   SOC - Current state of charge (0 to 100)
    % Outputs:
    %   LoadOn - Indicator if the load is on (1) or off (0)
    %   ChargingOn - Indicator if charging is active (1) or not (0)

    % Initialize persistent variables to retain state across function calls
    persistent LoadOnPersistent;
    persistent ChargingOnPersistent;

    if isempty(LoadOnPersistent)  % Initialize on first call
        LoadOnPersistent = 1;     % Load is initially on
        ChargingOnPersistent = 0;  % Charging is initially off
    end

    % Logic for charging and discharging based on SOC levels
    if SOC > 80
        LoadOnPersistent = 1;      % Turn load on if SOC is above 80%
        ChargingOnPersistent = 0;   % Turn charging off
    elseif SOC < 40
        LoadOnPersistent = 0;      % Turn load off if SOC is below 40%
        ChargingOnPersistent = 1;   % Start charging
    end

    % Assign output values from persistent variables
    LoadOn = LoadOnPersistent;
    ChargingOn = ChargingOnPersistent;
end
